simulink model "Practica1"  (R2023b)
settings: Solver=ode23  StartTime=0.0  StopTime=200  RelTol=1e-3
values from neighbouring files (symbols this model uses):
  g = 9.81    [Practica1.mat]
  l1 = 0.3    [Practica1.mat]
  l2 = 0.25    [Practica1.mat]
  m1 = 0.2    [Practica1.mat]
  m2 = 0.1    [Practica1.mat]

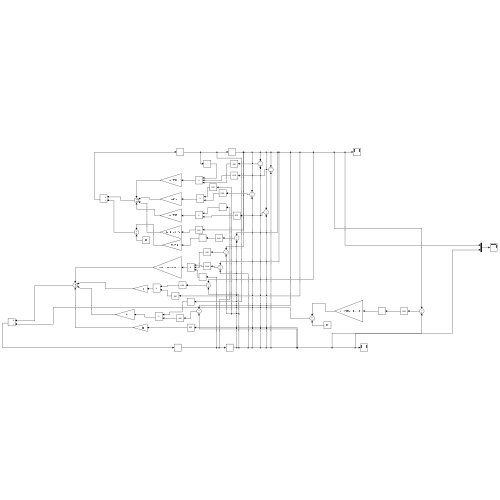
[thumbnail: Simulink's stored preview of the top-level diagram]
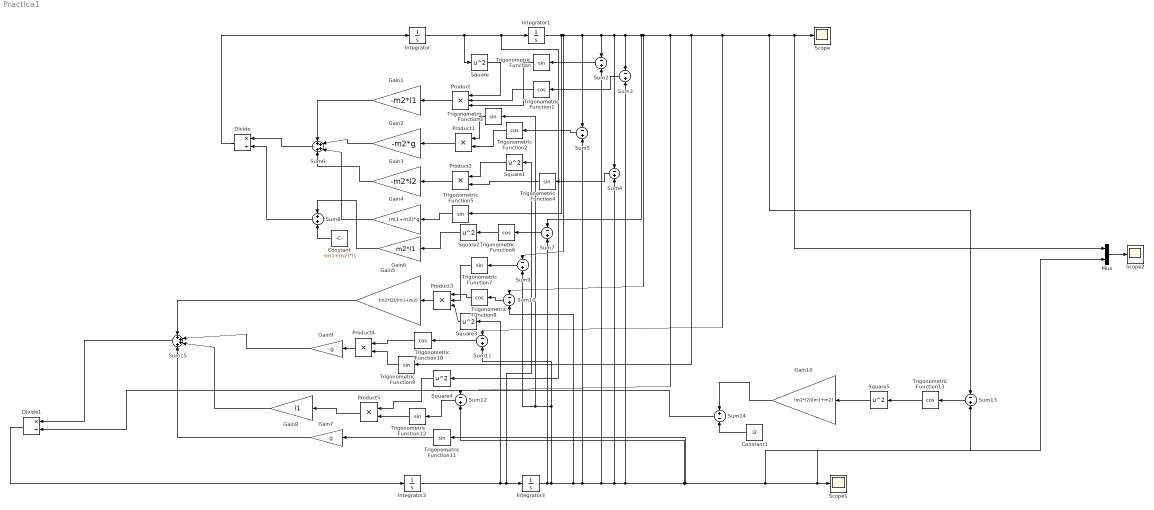
== system Practica1 ==
  Constant : Constant  Value=-(m1+m2)*l1
  Constant1 : Constant  Value=l2
  Divide : Product  Inputs=*/
  Divide1 : Product  Inputs=*/
  Gain1 : Gain  Gain=-m2*l1
  Gain10 : Gain  Gain=(m2*l2)/(m1+m2)
  Gain2 : Gain  Gain=-m2*g
  Gain3 : Gain  Gain=-m2*l2
  Gain4 : Gain  Gain=(m1+m2)*g
  Gain5 : Gain  Gain=(m2*l2)/(m1+m2)
  Gain6 : Gain  Gain=m2*l1
  Gain7 : Gain  Gain=g
  Gain8 : Gain  Gain=l1
  Gain9 : Gain  Gain=-g
  Integrator : Integrator
  Integrator1 : Integrator
  Integrator2 : Integrator
  Integrator3 : Integrator  InitialCondition=0.61086
  Mux : Mux  Inputs=2
  Product : Product  Inputs=3
  Product{1..2,4..5} (4 alike) : Product
  Product3 : Product  Inputs=3
  Scope : Scope
  Scope1 : Scope
  Scope2 : Scope
  Square{,1..5} (6 alike) : Math  Operator=square
  Sum{2..5,7,9..13} (10 alike) : Sum  Inputs=-+
  Sum14 : Sum  Inputs=+-
  Sum15 : Sum  Inputs=++++
  Sum6 : Sum  Inputs=++++
  Sum8 : Sum
  Trigonometric Function{,3..5,7,9,11..12} (8 alike) : Trigonometry
  Trigonometric Function{1..2,6,8,10,13} (6 alike) : Trigonometry  Operator=cos
  wires:
  Divide/1 -> Integrator/1
  Integrator/1 -> Square4/1, Integrator1/1, Square/1
  Square/1 -> Product/1
  Trigonometric Function/1 -> Product/3
  Divide1/1 -> Integrator2/1
  Integrator2/1 -> Square3/1, Square1/1, Integrator3/1
  Sum2/1 -> Trigonometric Function/1
  Sum3/1 -> Trigonometric Function1/1
  Trigonometric Function1/1 -> Product/2
  Product/1 -> Gain1/1
  Product1/1 -> Gain2/1
  Sum5/1 -> Trigonometric Function2/1
  Trigonometric Function3/1 -> Product1/1
  Trigonometric Function2/1 -> Product1/2
  Product2/1 -> Gain3/1
  Square1/1 -> Product2/1
  Sum4/1 -> Trigonometric Function4/1
  Trigonometric Function4/1 -> Product2/2
  Trigonometric Function5/1 -> Gain4/1
  Gain1/1 -> Sum6/1
  Gain2/1 -> Sum6/2
  Gain3/1 -> Sum6/4
  Gain4/1 -> Sum6/3
  Sum6/1 -> Divide/1
  Sum7/1 -> Trigonometric Function6/1
  Trigonometric Function6/1 -> Square2/1
  Square2/1 -> Gain6/1
  Gain6/1 -> Sum8/1
  Sum8/1 -> Divide/2
  Constant/1 -> Sum8/2
  Product3/1 -> Gain5/1
  Square3/1 -> Product3/3
  Sum9/1 -> Trigonometric Function7/1
  Trigonometric Function7/1 -> Product3/2
  Integrator3/1 -> Sum7/2, Sum11/2, Sum9/2, Trigonometric Function3/1, Sum13/2, Mux/2, Scope1/1, Trigonometric Function11/1, Sum12/2, Sum3/2, Sum4/2, Sum2/2, Sum5/2, Sum10/2
  Integrator1/1 -> Trigonometric Function5/1, Sum9/1, Sum7/1, Sum12/1, Trigonometric Function9/1, Sum13/1, Mux/1, Scope/1, Sum11/1, Sum10/1, Sum3/1, Sum4/1, Sum2/1, Sum5/1
  Sum10/1 -> Trigonometric Function8/1
  Trigonometric Function8/1 -> Product3/1
  Trigonometric Function9/1 -> Product4/2
  Trigonometric Function10/1 -> Product4/1
  Sum11/1 -> Trigonometric Function10/1
  Trigonometric Function11/1 -> Gain7/1
  Square4/1 -> Product5/1
  Product5/1 -> Gain8/1
  Trigonometric Function12/1 -> Product5/2
  Sum12/1 -> Trigonometric Function12/1
  Product4/1 -> Gain9/1
  Square5/1 -> Gain10/1
  Trigonometric Function13/1 -> Square5/1
  Sum13/1 -> Trigonometric Function13/1
  Gain10/1 -> Sum14/1
  Constant1/1 -> Sum14/2
  Gain5/1 -> Sum15/1
  Gain9/1 -> Sum15/2
  Gain8/1 -> Sum15/3
  Gain7/1 -> Sum15/4
  Sum15/1 -> Divide1/1
  Sum14/1 -> Divide1/2
  Mux/1 -> Scope2/1
